simulink model "BatteryDynamics"  (R2019b)
settings: Solver=FixedStepAuto  StartTime=0.0  StopTime=tfinal  FixedStep=1  RelTol=1e-3
InitFcn:
  | Init_Simulation;
StopFcn:
  | ECM_Data_Processing;
values from neighbouring files (symbols this model uses):
  A = [-1/(Rc*Cc), 1/(Rc*Cc) ... (first row only)    [Init_Simulation.m]    (also in Milosh_OL_Simulation.m = [   1,                0, 0, 0, 0, 0, 0; OL_Simulation.m = [   1,                0, 0, 0, 0, 0, 0; formQPMatrices_KronMethod.m = sys.A; generateElecModel.m = [0,         0)
  B = [1/Cc, 0 ... (first row only)    [Init_Simulation.m]    (also in Milosh_OL_Simulation.m = [                   -dt/Q; OL_Simulation.m = [                   -dt/Q; formQPMatrices_KronMethod.m = sys.B; generateElecModel.m = [ -1/(Q*3600))
  C = [1,0 ... (first row only)    [Init_Simulation.m]    (also in Milosh_OL_Simulation.m = [0, 0,   0, 1,      0,  0,      0; OL_Simulation.m = [0, 0,   0, 1,      0,  0,      0; formQPMatrices_KronMethod.m = sys.C; generateElecModel.m = zeros(1,2))
  C1 = tau./R1    [Init_Simulation.m]    (also in Milosh_OL_Simulation.m = tau/R1; OL_Simulation.m = tau/R1; generateElecModel.m = tau/R1)
  Q = mean(model.QParam)    [Init_Simulation.m]    (also in Milosh_OL_Simulation.m = getParamESC('QParam',25,model); OL_Simulation.m = getParamESC('QParam',25,model); formQPMatrices_KronMethod.m = penalty.Q; generateElecModel.m = getParamESC('QParam',Temp,model))
  R0 = model.R0Param    [Init_Simulation.m]    (also in Milosh_OL_Simulation.m = getParamESC('R0Param',25,model); OL_Simulation.m = getParamESC('R0Param',25,model); generateElecModel.m = getParamESC('R0Param',Temp,model))
  R1 = model.RParam    [Init_Simulation.m]    (also in Milosh_OL_Simulation.m = getParamESC('RParam',25,model); OL_Simulation.m = getParamESC('RParam',25,model); generateElecModel.m = getParamESC('RParam',Temp,model))
  set_profile = 0    [Init_Simulation.m]
  Tamb = 25    [Init_Simulation.m]
  Tc0 = 25    [Init_Simulation.m]
  temperatures = model.temps    [Init_Simulation.m]
  Ts0 = 25    [Init_Simulation.m]
  Vc0 = 0    [Init_Simulation.m]
  z0 = 0.5    [Init_Simulation.m]
undefined symbols (not defined in the file or in its folder): model
settings Model: Creator=miloshstojcic  LastModifiedBy=miloshstojcic

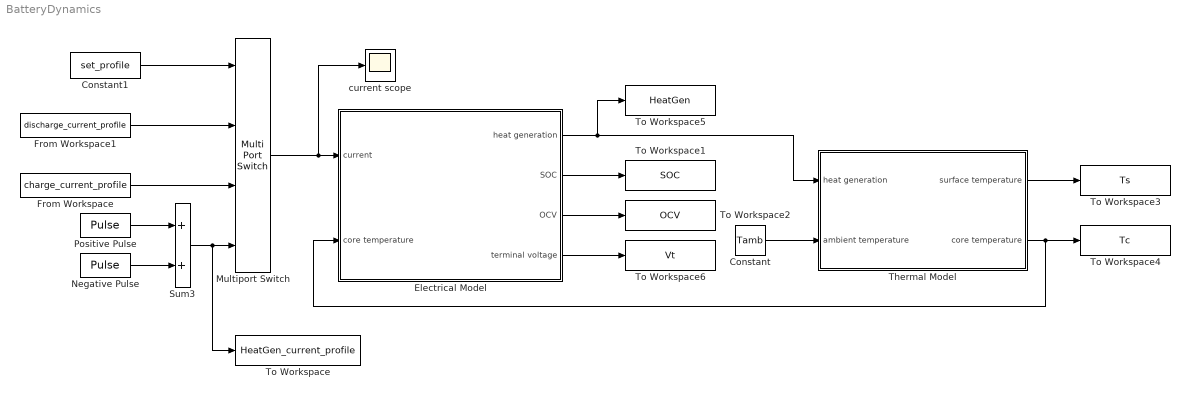
== system BatteryDynamics ==
  Constant : Constant  Value=Tamb
  Constant1 : Constant  Value=set_profile
  Electrical Model : Subsystem
  From Workspace : FromWorkspace  VariableName=charge_current_profile  SampleTime=0
  From Workspace1 : FromWorkspace  VariableName=discharge_current_profile  SampleTime=0
  Multiport Switch : MultiPortSwitch  DataPortOrder=Zero-based contiguous  zeroidx=on
  Negative Pulse : DiscretePulseGenerator  PulseType=Time based  Amplitude=-2.5*Q  Period=20  PulseWidth=50  PhaseDelay=10
  Positive Pulse : DiscretePulseGenerator  PulseType=Time based  Amplitude=2.5*Q  Period=20  PulseWidth=50
  Sum3 : Sum
  Thermal Model : Subsystem
  To Workspace : ToWorkspace  VariableName=HeatGen_current_profile  SampleTime=-1
      settings: Save2DSignal=2-D array (concatenate along first dimension)
  To Workspace1 : ToWorkspace  VariableName=SOC  SampleTime=-1
      settings: Save2DSignal=2-D array (concatenate along first dimension)
  To Workspace2 : ToWorkspace  VariableName=OCV  SampleTime=-1
      settings: Save2DSignal=2-D array (concatenate along first dimension)
  To Workspace3 : ToWorkspace  VariableName=Ts  SampleTime=-1
      settings: Save2DSignal=2-D array (concatenate along first dimension)
  To Workspace4 : ToWorkspace  VariableName=Tc  SampleTime=-1
      settings: Save2DSignal=2-D array (concatenate along first dimension)
  To Workspace5 : ToWorkspace  VariableName=HeatGen  SampleTime=-1
      settings: Save2DSignal=2-D array (concatenate along first dimension)
  To Workspace6 : ToWorkspace  VariableName=Vt  SampleTime=-1
      settings: Save2DSignal=2-D array (concatenate along first dimension)
  current scope : Scope
  wires:
  Thermal Model/2(core temperature) -> To Workspace4/1, Electrical Model/2(core temperature)
  Electrical Model/2(SOC) -> To Workspace1/1
  Electrical Model/3(OCV) -> To Workspace2/1
  Electrical Model/4(terminal voltage) -> To Workspace6/1
  Constant/1 -> Thermal Model/2(ambient temperature)
  Electrical Model/1(heat generation) -> To Workspace5/1, Thermal Model/1(heat generation)
  Thermal Model/1(surface temperature) -> To Workspace3/1
  Negative Pulse/1 -> Sum3/2
  Positive Pulse/1 -> Sum3/1
  Sum3/1 -> To Workspace/1, Multiport Switch/4
  From Workspace1/1 -> Multiport Switch/2
  Multiport Switch/1 -> current scope/1, Electrical Model/1(current)
  Constant1/1 -> Multiport Switch/1
  From Workspace/1 -> Multiport Switch/3

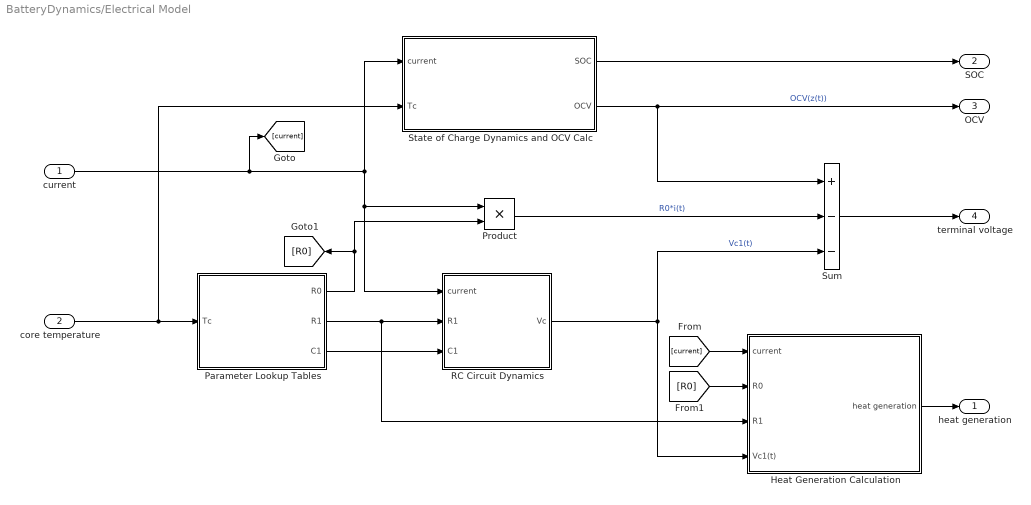
== system BatteryDynamics/Electrical Model ==
  current : Inport
  core temperature : Inport  Port=2
  Heat Generation Calculation : Subsystem
  Parameter Lookup Tables : Subsystem
  Product : Product
  RC Circuit Dynamics : Subsystem
  State of Charge Dynamics and OCV Calc : Subsystem
  Sum : Sum  Inputs=+--
  heat generation : Outport
  SOC : Outport  Port=2
  OCV : Outport  Port=3
  terminal voltage : Outport  Port=4
  wires:
  Sum/1 -> terminal voltage/1
  State of Charge Dynamics and OCV Calc/1(SOC) -> SOC/1
  Parameter Lookup Tables/3(C1) -> RC Circuit Dynamics/3(C1)
  core temperature/1 -> State of Charge Dynamics and OCV Calc/2(Tc), Parameter Lookup Tables/1(Tc)
  RC Circuit Dynamics/1(Vc) -> Heat Generation Calculation/4(Vc1(t)), Sum/3  "Vc1(t)"
  Parameter Lookup Tables/2(R1) -> Heat Generation Calculation/3(R1), RC Circuit Dynamics/2(R1)
  State of Charge Dynamics and OCV Calc/2(OCV) -> OCV/1, Sum/1  "OCV(z(t))"
  current/1 -> [current], State of Charge Dynamics and OCV Calc/1(current), Product/1, RC Circuit Dynamics/1(current)
  Product/1 -> Sum/2  "R0*i(t)"
  Parameter Lookup Tables/1(R0) -> Product/2, [R0]
  Heat Generation Calculation/1(heat generation) -> heat generation/1
  [current] -> Heat Generation Calculation/1(current)
  [R0] -> Heat Generation Calculation/2(R0)

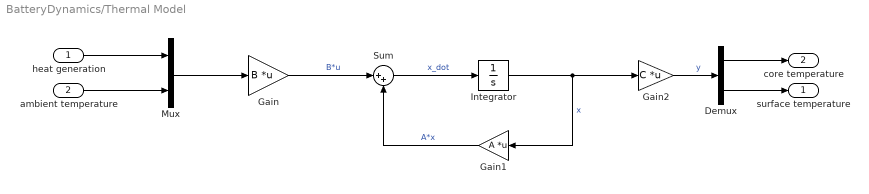
== system BatteryDynamics/Thermal Model ==
  heat generation : Inport
  ambient temperature : Inport  Port=2
  Demux : Demux  Outputs=2
  Gain : Gain  Gain=B  Multiplication=Matrix(K*u)
  Gain1 : Gain  Gain=A  Multiplication=Matrix(K*u)
  Gain2 : Gain  Gain=C  Multiplication=Matrix(K*u)
  Integrator : Integrator  InitialCondition=[Tc0;Ts0]
  Mux : Mux  Inputs=2
  Sum : Sum  Inputs=|++
  surface temperature : Outport
  core temperature : Outport  Port=2
  wires:
  ambient temperature/1 -> Mux/2
  heat generation/1 -> Mux/1
  Mux/1 -> Gain/1
  Gain/1 -> Sum/1  "B*u"
  Sum/1 -> Integrator/1  "x_dot"
  Gain1/1 -> Sum/2  "A*x"
  Integrator/1 -> Gain2/1, Gain1/1  "x"
  Gain2/1 -> Demux/1  "y"
  Demux/2 -> surface temperature/1
  Demux/1 -> core temperature/1

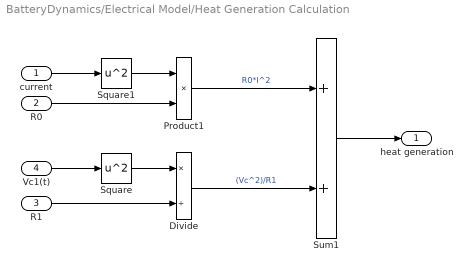
== system BatteryDynamics/Electrical Model/Heat Generation Calculation ==
  current : Inport
  R0 : Inport  Port=2
  R1 : Inport  Port=3
  Vc1(t) : Inport  Port=4
  Divide : Product  Inputs=*/
  Product1 : Product
  Square : Math  Operator=square  SignedPower=off  SaturateOnIntegerOverflow=on
  Square1 : Math  Operator=square  SignedPower=off  SaturateOnIntegerOverflow=on
  Sum1 : Sum
  heat generation : Outport
  wires:
  Vc1(t)/1 -> Square/1
  current/1 -> Square1/1
  Square/1 -> Divide/1
  R0/1 -> Product1/2
  Square1/1 -> Product1/1
  Sum1/1 -> heat generation/1
  R1/1 -> Divide/2
  Product1/1 -> Sum1/1  "R0*I^2"
  Divide/1 -> Sum1/2  "(Vc^2)/R1"

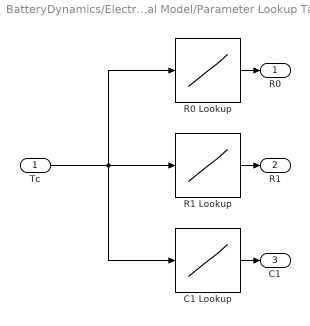
== system BatteryDynamics/Electrical Model/Parameter Lookup Tables ==
  Tc : Inport
  C1 Lookup : Lookup_n-D  NumberOfTableDimensions=1  BreakpointsForDimension1=temperatures  BreakpointsForDimension1FirstPoint=temperatures(1)  Table=C1  InternalRulePriority=Speed  RndMeth=Simplest  InputSameDT=on
  R0 Lookup : Lookup_n-D  NumberOfTableDimensions=1  BreakpointsForDimension1=temperatures  BreakpointsForDimension1FirstPoint=temperatures(1)  Table=R0  InternalRulePriority=Speed  RndMeth=Simplest  InputSameDT=on
  R1 Lookup : Lookup_n-D  NumberOfTableDimensions=1  BreakpointsForDimension1=temperatures  BreakpointsForDimension1FirstPoint=temperatures(1)  Table=R1  InternalRulePriority=Speed  RndMeth=Simplest  InputSameDT=on
  R0 : Outport
  R1 : Outport  Port=2
  C1 : Outport  Port=3
  wires:
  R0 Lookup/1 -> R0/1
  R1 Lookup/1 -> R1/1
  C1 Lookup/1 -> C1/1
  Tc/1 -> R0 Lookup/1, R1 Lookup/1, C1 Lookup/1

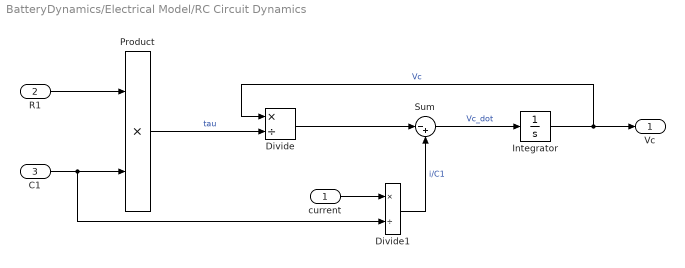
== system BatteryDynamics/Electrical Model/RC Circuit Dynamics ==
  current : Inport
  R1 : Inport  Port=2
  C1 : Inport  Port=3
  Divide : Product  Inputs=*/
  Divide1 : Product  Inputs=*/
  Integrator : Integrator  InitialCondition=Vc0
  Product : Product
  Sum : Sum  Inputs=|-+
  Vc : Outport
  wires:
  C1/1 -> Divide1/2, Product/2
  R1/1 -> Product/1
  current/1 -> Divide1/1
  Divide1/1 -> Sum/2  "i/C1"
  Sum/1 -> Integrator/1  "Vc_dot"
  Integrator/1 -> Divide/1, Vc/1  "Vc"
  Product/1 -> Divide/2  "tau"
  Divide/1 -> Sum/1

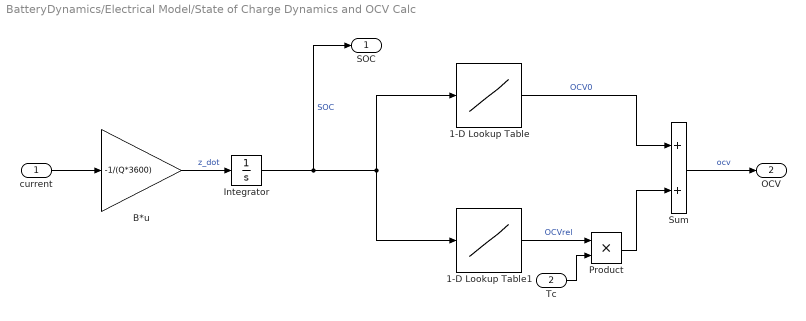
== system BatteryDynamics/Electrical Model/State of Charge Dynamics and OCV Calc ==
  current : Inport
  Tc : Inport  Port=2
  1-D Lookup Table : Lookup_n-D  NumberOfTableDimensions=1  BreakpointsForDimension1=0:0.005:1  BreakpointsForDimension1FirstPoint=0  Table=model.OCV0  InternalRulePriority=Speed  RndMeth=Simplest  InputSameDT=on
  1-D Lookup Table1 : Lookup_n-D  NumberOfTableDimensions=1  BreakpointsForDimension1=[0:0.005:1]  BreakpointsForDimension1FirstPoint=0  Table=model.OCVrel  InternalRulePriority=Speed  RndMeth=Simplest  InputSameDT=on
  B*u : Gain  Gain=-1/(Q*3600)
  Integrator : Integrator  InitialCondition=z0
  Product : Product
  Sum : Sum
  SOC : Outport
  OCV : Outport  Port=2
  wires:
  current/1 -> B*u/1
  Sum/1 -> OCV/1  "ocv"
  B*u/1 -> Integrator/1  "z_dot"
  1-D Lookup Table1/1 -> Product/1  "OCVrel"
  Product/1 -> Sum/2
  1-D Lookup Table/1 -> Sum/1  "OCV0"
  Integrator/1 -> SOC/1, 1-D Lookup Table1/1, 1-D Lookup Table/1  "SOC"
  Tc/1 -> Product/2
